simulink model "Zimpedence_SZ_design_V1_0"  (R2017b)
settings: Solver=ode45  StartTime=0.0  StopTime=0.1  MaxStep=1e-6  RelTol=1e-3
InitFcn:
  | clear;
  | clc;
  | format long;
  | f = 85e3;
  | w = 2*pi*f;
undefined symbols (not defined in the file): Cz, Lp, Lz
libraries: powerlib x17, simulink x4, peRmsMeasurement x4, powerlib_meascontrol x4
settings Model: Creator=SuperWindows  LastModifiedBy=SuperWindows
settings DebuggingCC: UnconnectedInputMsg=none  UnconnectedOutputMsg=none  UnconnectedLineMsg=none

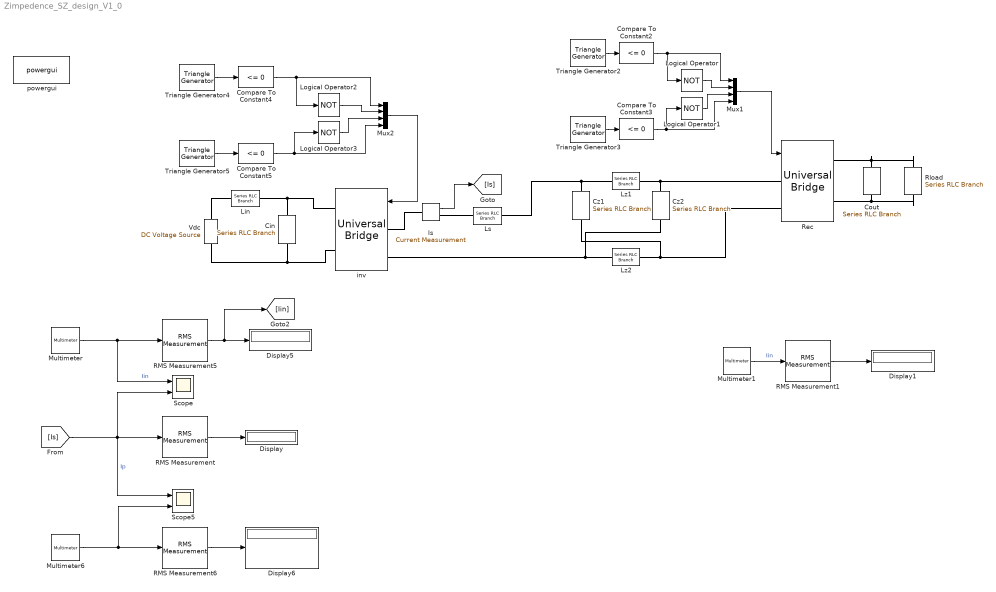
== system Zimpedence_SZ_design_V1_0 ==
  Cin : powerlib/Elements/Series RLC Branch  LConnTagsString=__new0  RConnTagsString=__new0  BranchType=RC  Resistance=0.1  Inductance=Lz  SetiL0=off  InitialCurrent=0  Capacitance=10e-6  Setx0=off  InitialVoltage=0  Measurements=Branch voltage and current
  Compare To Constant{2..5} (4 alike) : simulink/Logic and Bit Operations/Compare To Constant  relop=<=  const=0  OutDataTypeStr=boolean
  Cout : powerlib/Elements/Series RLC Branch  LConnTagsString=__new0  RConnTagsString=__new0  BranchType=C  Resistance=1  Inductance=Lp  SetiL0=off  InitialCurrent=0  Capacitance=470e-6  Setx0=on  InitialVoltage=90  Measurements=Branch voltage and current
  Cz1 : powerlib/Elements/Series RLC Branch  LConnTagsString=__new0  RConnTagsString=__new0  BranchType=C  Resistance=1  Inductance=Lp  SetiL0=off  InitialCurrent=0  Capacitance=82.37e-9  Setx0=off  InitialVoltage=0  Measurements=Branch voltage and current
  Cz2 : powerlib/Elements/Series RLC Branch  LConnTagsString=__new0  RConnTagsString=__new0  BranchType=C  Resistance=1  Inductance=Lp  SetiL0=off  InitialCurrent=0  Capacitance=82.15e-9  Setx0=off  InitialVoltage=0  Measurements=Branch voltage and current
  Display{,1,5..6} (4 alike) : Display
  Is : powerlib/Measurements/Current Measurement  PhasorSimulation=off  OutputType=Complex  PSBequivalent=0
  Lin : powerlib/Elements/Series RLC Branch  LConnTagsString=__new0  RConnTagsString=__new0  BranchType=L  Resistance=1  Inductance=10e-6  SetiL0=off  InitialCurrent=0  Capacitance=Cz  Setx0=off  InitialVoltage=0  Measurements=Branch voltage and current
  Logical Operator{,1..3} (4 alike) : Logic  Operator=NOT  AllPortsSameDT=off  OutDataTypeStr=boolean
  Ls : powerlib/Elements/Series RLC Branch  LConnTagsString=__new0  RConnTagsString=__new0  BranchType=RL  Resistance=275e-3  Inductance=289.05e-6  SetiL0=off  InitialCurrent=0  Capacitance=Cz  Setx0=off  InitialVoltage=0  Measurements=Branch voltage and current
  Lz1 : powerlib/Elements/Series RLC Branch  LConnTagsString=__new0  RConnTagsString=__new0  BranchType=RL  Resistance=48.6e-3  Inductance=66.76e-6  SetiL0=off  InitialCurrent=0  Capacitance=Cz  Setx0=off  InitialVoltage=0  Measurements=Branch voltage and current
  Lz2 : powerlib/Elements/Series RLC Branch  LConnTagsString=__new0  RConnTagsString=__new0  BranchType=RL  Resistance=43.7e-3  Inductance=66.97e-6  SetiL0=off  InitialCurrent=0  Capacitance=Cz  Setx0=off  InitialVoltage=0  Measurements=Branch voltage and current
  Multimeter : powerlib/Measurements/Multimeter  PhasorSimulation=off  OutputType=Complex  sel=26  L=38  Gain=1  yselected={'Ib: Lin'};  PSBOutputType=1  PSBequivalent=0  AxesSetting=[0,0.1,-100,100]  Display=0  SavedBlockNames=-11
  Multimeter1 : powerlib/Measurements/Multimeter  PhasorSimulation=off  OutputType=Complex  sel=8  L=38  Gain=1  yselected={'Ub: Rload'};  PSBOutputType=1  PSBequivalent=0  AxesSetting=[0,0.1,-100,100]  Display=0  SavedBlockNames=-11
  Multimeter6 : powerlib/Measurements/Multimeter  PhasorSimulation=off  OutputType=Complex  sel=14  L=38  Gain=1  yselected={'Uab: inv'};  PSBOutputType=1  PSBequivalent=0  AxesSetting=[0,0.1,-100,100]  Display=0  SavedBlockNames=-11
  Mux1 : Mux
  Mux2 : Mux
  RMS Measurement : peRmsMeasurement/RMS Measurement  OverrideUsingVariant=Total  F=f  SpecifyHarmonics=off  K=[0 1 2]  Ts=0
  RMS Measurement1 : peRmsMeasurement/RMS Measurement  OverrideUsingVariant=Total  F=f/10  SpecifyHarmonics=off  K=[0 1 2]  Ts=0
  RMS Measurement5 : peRmsMeasurement/RMS Measurement  OverrideUsingVariant=Total  F=f/10  SpecifyHarmonics=off  K=[0 1 2]  Ts=0
  RMS Measurement6 : peRmsMeasurement/RMS Measurement  OverrideUsingVariant=Harmonic  F=f  SpecifyHarmonics=on  K=[0 1 2]  Ts=0
  Rec : powerlib/Power Electronics/Universal Bridge  Arms=2  SnubberResistance=1e5  SnubberCapacitance=inf  Device=MOSFET / Diodes  Ron=80e-3  Lon=0  ForwardVoltages="[  0  0  ]"  ForwardVoltage=0.45  GTOparameters=[ 10e-6 , 20e-6 ]  IGBTparameters=[ 1e-6 , 2e-6 ]  Measurements=All voltages and currents  Measurements_2=None  converterType=Rectifier
  Rload : powerlib/Elements/Series RLC Branch  LConnTagsString=__new0  RConnTagsString=__new0  BranchType=R  Resistance=6.17  Inductance=Lp  SetiL0=off  InitialCurrent=0  Capacitance=470e-6  Setx0=off  InitialVoltage=0  Measurements=Branch voltage and current
  Scope : Scope  NumInputPorts=2
  Scope5 : Scope  NumInputPorts=2
  Triangle Generator{2..5} (4 alike) : powerlib_meascontrol/Pulse & Signal Generators/Triangle Generator  Freq=f  Phase=0  Ts=0
  Vdc : powerlib/Electrical Sources/DC Voltage Source  Amplitude=50  Measurements=None
  inv : powerlib/Power Electronics/Universal Bridge  Arms=2  SnubberResistance=1e5  SnubberCapacitance=inf  Device=MOSFET / Diodes  Ron=80e-3  Lon=0  ForwardVoltages="[  0  0  ]"  ForwardVoltage=0  GTOparameters=[ 10e-6 , 20e-6 ]  IGBTparameters=[ 1e-6 , 2e-6 ]  Measurements=All voltages and currents  Measurements_2=None  converterType=Rectifier
  powergui : powerlib/powergui  Priority=1  SimulationMode=Discrete  SampleTime=5e-8  frequency=60  Iterations=50  frequencyindice=0  Pbase=100e6  ErrMax=1e-4  UnitsV=kV  UnitsW=MW  buscounter=0  FunctionMessages=off  echomessages=off  EnableUseOfTLC=off  CurrentSourceSwitches=off  DisableSnubberDevices=off  DisableRonSwitches=off  DisableVfSwitches=off  DisplayEquations=off  SolverType=Tustin/Backward Euler (TBE)  Interpol=off  ExternalGateDelay=off  methode=off  Ts=100  x0status=blocks  SPID=on  SwTol=0  HookPort=off  RestoreLinks=warning  ResistiveCurrentMeasurement=off  Frange=[0:2:500]  Ylog=off  Xlog=on  ShowGrid=off  save=off  variable=ZData  structure=ULZ  ZoomFFT=off  StartTime=0.03135  cycles=30  DisplayStyle=2  fundamental=85e3  FreqAxis=off  MaxFrequency=100*85e3  frequencyindicesteady=1  RmsSteady=1  display=off
  wires:
  Compare To Constant2/1 -> Mux1/1, Logical Operator/1
  Triangle Generator3/1 -> Compare To Constant3/1
  Compare To Constant3/1 -> Mux1/4, Logical Operator1/1
  Triangle Generator2/1 -> Compare To Constant2/1
  Logical Operator1/1 -> Mux1/3
  Logical Operator/1 -> Mux1/2
  Logical Operator2/1 -> Mux2/2
  Logical Operator3/1 -> Mux2/3
  Triangle Generator4/1 -> Compare To Constant4/1
  Triangle Generator5/1 -> Compare To Constant5/1
  Compare To Constant5/1 -> Mux2/4, Logical Operator3/1
  Compare To Constant4/1 -> Mux2/1, Logical Operator2/1
  Mux2/1 -> inv/1
  [Is] -> Scope/2, Scope5/1, RMS Measurement/1  "Ip"
  Multimeter/1 -> Scope/1, RMS Measurement5/1  "Iin"
  RMS Measurement5/1 -> [Iin], Display5/1
  Multimeter6/1 -> Scope5/2, RMS Measurement6/1
  Mux1/1 -> Rec/1
  RMS Measurement/1 -> Display/1
  RMS Measurement6/1 -> Display6/1
  Is/1 -> [Is]
  Multimeter1/1 -> RMS Measurement1/1  "Iin"
  RMS Measurement1/1 -> Display1/1
  connections:
  Vdc/LConn1 -- Cin/RConn1 -- inv/RConn2
  Lz1/LConn1 -- Ls/RConn1 -- Cz1/LConn1
  Cz2/RConn1 -- Lz2/LConn1 -- inv/LConn2
  Lz2/RConn1 -- Rec/LConn2 -- Cz1/RConn1
  Cout/LConn1 -- Rload/LConn1 -- Rec/RConn1
  Rload/RConn1 -- Rec/RConn2 -- Cout/RConn1
  Lin/LConn1 -- Vdc/RConn1
  Lin/RConn1 -- Cin/LConn1 -- inv/RConn1
  Lz1/RConn1 -- Rec/LConn1 -- Cz2/LConn1
  Is/LConn1 -- inv/LConn1
  Is/RConn1 -- Ls/LConn1
